simulink model "gm_uz_pmsm_model"  (R2023b)
settings: Solver=FixedStepAuto  StartTime=0.0  StopTime=0.05  RelTol=1e-3
PreLoadFcn:
  | uz_pmsm_model_init_parameter
PostLoadFcn:
  | % Import the data from Excel for a lookup table
  | FluxMapData = readtable('C:\Users\Philipp\ultrazohm\ultrazohm_sw\ip_cores\uz_pmsm_model\FluxMapData_2023-05-26_13-07-57.csv');
  | % Row indices for lookup table
  | d_current_in_d_axis = FluxMapData(8:27,1:end);
  | % Column indices for lookup table
  | q_current_in_d_axis = FluxMapData(29:48,1:end);
  | % Output values for lookup table
  | d_Flux_d_axis = FluxMapData(50:69,1:end);
undefined symbols (not defined in the file or in its folder): ad1, ad2, ad3, ad4, ad5, ad6, aq1, aq2, aq3, aq4, aq5, aq6, d_current_d_Flux, d_current_q_Flux, entkopplung_dynamic, entkopplung_linear, entkopplung_static, Fid1_Giq1, Fid2_Giq2, Flux_d, Flux_q, friction_coefficient, inertia, Ki_Bo_d, Ki_Bo_q, Kp_Bo_d, Kp_Bo_q, L_d, L_q, Ldq, parameter_nachfuerung, polepair, praediktion_entkopplung_nonlinear, psi_pm, q_current_d_Flux, q_current_q_Flux, R_1, simulate_mechanical, simulate_nonlinear_modell, simulate_open_loop, static_friction_torque, tau_sum, ts_regler
libraries: hdlmdlgenlib x21, slpidlib x6
(part 3 of 4)

== system gm_uz_pmsm_model/Current_Controller1/Entkopplungen ==
  u_q : Inport
  u_d : Inport  Port=2
  uq : Inport  Port=3
  ud : Inport  Port=4
  i_d : Inport  Port=5
  psi_d_LUT : Inport  Port=6
  psi_q_LUT : Inport  Port=7
  Ldq_LUT : Inport  Port=8
  Lqd_LUT : Inport  Port=9
  i_q : Inport  Port=10
  omega_m : Inport  Port=11
  Lineare_Entkopplung : Subsystem
  decoupling_praediktion : Subsystem
  dynamic_nonlinear_entkopplung1 : Subsystem  Commented=on
  static_nonlinear_entkopplung : Subsystem
  u_d_static : Outport
  u_q_static : Outport  Port=2
  u_d_prae : Outport  Port=3
  u_q_prae : Outport  Port=4
  u_d_lin : Outport  Port=5
  u_q_lin : Outport  Port=6
  u_d_dyn : Outport  Port=7
  u_q_dyn1 : Outport  Port=8
  wires:
  Lqd_LUT/1 -> dynamic_nonlinear_entkopplung1/6(Lqd_LUT)
  Ldq_LUT/1 -> dynamic_nonlinear_entkopplung1/5(Ldq_LUT)
  dynamic_nonlinear_entkopplung1/2(u_q) -> u_q_dyn1/1
  dynamic_nonlinear_entkopplung1/1(u_d) -> u_d_dyn/1
  decoupling_praediktion/2(u_q_entk) -> u_q_prae/1
  Lineare_Entkopplung/2(u_q) -> u_q_lin/1
  decoupling_praediktion/1(u_d_entk) -> u_d_prae/1
  static_nonlinear_entkopplung/2(u_q) -> u_q_static/1
  Lineare_Entkopplung/1(u_d) -> u_d_lin/1
  static_nonlinear_entkopplung/1(u_d) -> u_d_static/1
  u_d/1 -> decoupling_praediktion/2(u_d_1)
  uq/1 -> decoupling_praediktion/7(u_q_k)
  ud/1 -> decoupling_praediktion/6(u_d_k)
  i_q/1 -> decoupling_praediktion/3(i_q), Lineare_Entkopplung/2(i_q), dynamic_nonlinear_entkopplung1/2(i_q)
  i_d/1 -> decoupling_praediktion/1(i_d), Lineare_Entkopplung/1(i_d), dynamic_nonlinear_entkopplung1/1(i_d)
  u_q/1 -> decoupling_praediktion/4(u_q_1)
  psi_q_LUT/1 -> static_nonlinear_entkopplung/2(psi_q), decoupling_praediktion/8(psi_q), dynamic_nonlinear_entkopplung1/4(psi_q)
  omega_m/1 -> decoupling_praediktion/5(omega_m), static_nonlinear_entkopplung/3(omega_m), Lineare_Entkopplung/3(omega_m), dynamic_nonlinear_entkopplung1/7(omega_m)
  psi_d_LUT/1 -> decoupling_praediktion/9(psi_d), dynamic_nonlinear_entkopplung1/3(psi_d), static_nonlinear_entkopplung/1(psi_d)

== system gm_uz_pmsm_model/Current_Controller1/Psi_d_q1 ==
  I_d : Inport
  I_q : Inport  Port=2
  ApproxPara : Inport  Port=3
  Ldd_approx1 : Subsystem
  Lqq_approx1 : Subsystem
  psid_approx : Subsystem
  psiq_approx : Subsystem
  psi_d : Outport
  Ldd : Outport  Port=2
  psi_q : Outport  Port=3
  Lqq : Outport  Port=4
  wires:
  ApproxPara/1 -> Lqq_approx1/3(FittingParameters), psid_approx/3(FittingParameters), Ldd_approx1/3(FittingParameters), psiq_approx/3(FittingParameters)
  Lqq_approx1/1(Lqq) -> Lqq/1  "Lqq"
  Ldd_approx1/1(Ldd) -> Ldd/1  "Ldd"
  psiq_approx/2(psid_cross_s1_integrated) -> Lqq_approx1/1(psid_cross_s1_integrated)
  I_d/1 -> psiq_approx/1(Id), psid_approx/1(Id), Ldd_approx1/2(Id)
  psid_approx/2(psiq_cross_s1_integrated) -> Ldd_approx1/1(psiq_cross_s1_integrated)
  I_q/1 -> psiq_approx/2(Iq), Lqq_approx1/2(Iq), psid_approx/2(Iq)
  psiq_approx/1(psiq) -> psi_q/1  "psi_q"
  psid_approx/1(psid) -> psi_d/1  "psi_d"

== system gm_uz_pmsm_model/Current_Controller1/Reglernachführung ==
  Flag : Inport
  Ldd : Inport  Port=2
  Lqq : Inport  Port=3
  Constant : Constant  Value=1/(2*tau_sum)
  Constant1 : Constant  Value=R_1
  Constant2 : Constant  Value=L_d
  Constant3 : Constant  Value=L_q
  Product : Product
  Product1 : Product
  Product2 : Product
  Rate Transition1 : RateTransition  OutPortSampleTime=ts_regler
  Rate Transition12 : RateTransition  OutPortSampleTime=ts_regler
  Switch : Switch  Criteria=u2 > Threshold  SaturateOnIntegerOverflow=off  InputSameDT=off  OutDataTypeStr=Inherit: Same as first input
  Switch1 : Switch  Criteria=u2 > Threshold  SaturateOnIntegerOverflow=off  InputSameDT=off  OutDataTypeStr=Inherit: Same as first input
  K_p_d : Outport
  K_p_q : Outport  Port=2
  K_I : Outport  Port=3
  wires:
  Constant1/1 -> Rate Transition1/1  "u_q"
  Lqq/1 -> Switch1/1  "Lqq"
  Ldd/1 -> Switch/1  "Ldd"
  Switch1/1 -> Product1/2
  Constant3/1 -> Switch1/3
  Switch/1 -> Product/1
  Constant2/1 -> Switch/3
  Flag/1 -> Switch1/2, Switch/2
  Rate Transition1/1 -> Product2/2  "id_regler"
  Rate Transition12/1 -> Product/2, Product1/1, Product2/1  "id_regler"
  Product2/1 -> K_I/1
  Product1/1 -> K_p_q/1
  Product/1 -> K_p_d/1
  Constant/1 -> Rate Transition12/1

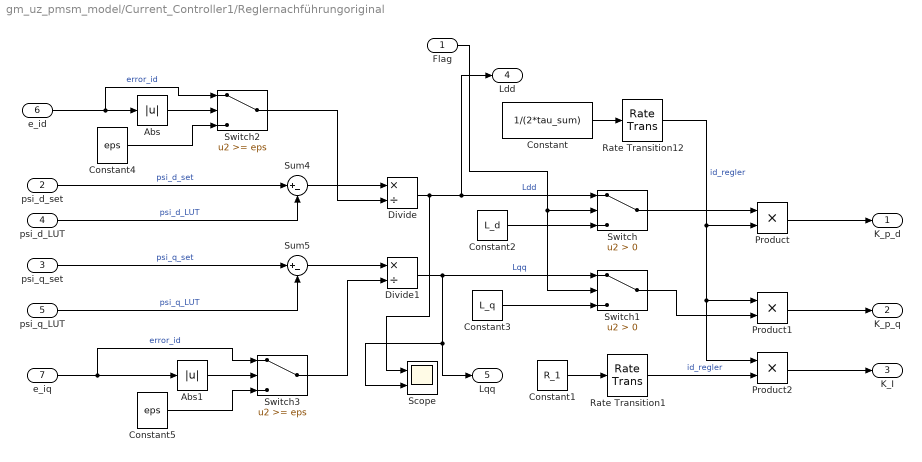
== system gm_uz_pmsm_model/Current_Controller1/Reglernachführungoriginal ==
  Flag : Inport
  psi_d_set : Inport  Port=2
  psi_q_set : Inport  Port=3
  psi_d_LUT : Inport  Port=4
  psi_q_LUT : Inport  Port=5
  e_id : Inport  Port=6
  e_iq : Inport  Port=7
  Abs : Abs  SaturateOnIntegerOverflow=off
  Abs1 : Abs  SaturateOnIntegerOverflow=off
  Constant : Constant  Value=1/(2*tau_sum)
  Constant1 : Constant  Value=R_1
  Constant2 : Constant  Value=L_d
  Constant3 : Constant  Value=L_q
  Constant4 : Constant  Value=eps  SampleTime=ts_regler
  Constant5 : Constant  Value=eps  SampleTime=ts_regler
  Divide : Product  Inputs=*/
  Divide1 : Product  Inputs=*/
  Product : Product
  Product1 : Product
  Product2 : Product
  Rate Transition1 : RateTransition  OutPortSampleTime=ts_regler
  Rate Transition12 : RateTransition  OutPortSampleTime=ts_regler
  Scope : Scope  NumInputPorts=2
  Sum4 : Sum  Inputs=|+-
  Sum5 : Sum  Inputs=|+-
  Switch : Switch  Criteria=u2 > Threshold  SaturateOnIntegerOverflow=off  InputSameDT=off
  Switch1 : Switch  Criteria=u2 > Threshold  SaturateOnIntegerOverflow=off  InputSameDT=off
  Switch2 : Switch  Threshold=eps  SaturateOnIntegerOverflow=off  InputSameDT=off
  Switch3 : Switch  Threshold=eps  SaturateOnIntegerOverflow=off  InputSameDT=off
  K_p_d : Outport
  K_p_q : Outport  Port=2
  K_I : Outport  Port=3
  Ldd : Outport  Port=4
  Lqq : Outport  Port=5
  wires:
  Constant5/1 -> Switch3/3
  Abs1/1 -> Switch3/2
  Switch3/1 -> Divide1/2
  e_iq/1 -> Abs1/1, Switch3/1  "error_id"
  Switch2/1 -> Divide/2
  Abs/1 -> Switch2/2
  Constant4/1 -> Switch2/3
  e_id/1 -> Abs/1, Switch2/1  "error_id"
  Divide1/1 -> Switch1/1, Lqq/1, Scope/2  "Lqq"
  Divide/1 -> Switch/1, Ldd/1, Scope/1  "Ldd"
  psi_q_set/1 -> Sum5/1  "psi_q_set"
  psi_d_set/1 -> Sum4/1  "psi_d_set"
  psi_d_LUT/1 -> Sum4/2  "psi_d_LUT"
  Sum5/1 -> Divide1/1
  psi_q_LUT/1 -> Sum5/2  "psi_q_LUT"
  Sum4/1 -> Divide/1
  Switch1/1 -> Product1/2
  Constant3/1 -> Switch1/3
  Switch/1 -> Product/1
  Constant2/1 -> Switch/3
  Flag/1 -> Switch1/2, Switch/2
  Rate Transition1/1 -> Product2/2  "id_regler"
  Rate Transition12/1 -> Product/2, Product1/1, Product2/1  "id_regler"
  Constant1/1 -> Rate Transition1/1
  Product2/1 -> K_I/1
  Product1/1 -> K_p_q/1
  Product/1 -> K_p_d/1
  Constant/1 -> Rate Transition12/1

== system gm_uz_pmsm_model/Current_Controller_With_FluxMaps_OLD1/Entkopplung_flags ==
  u_d_static : Inport
  u_q_static : Inport  Port=2
  u_d_praed : Inport  Port=3
  u_q_praed : Inport  Port=4
  u_d_lin : Inport  Port=5
  u_q_lin : Inport  Port=6
  u_d_dyn : Inport  Port=7
  u_q_dyn : Inport  Port=8
  0 : Constant  Value=0
  Switch{1..8} (8 alike) : Switch  Criteria=u2 > Threshold  SaturateOnIntegerOverflow=off  InputSameDT=off
  entkopplung_dynamic : Constant  Value=entkopplung_dynamic
  entkopplung_linear : Constant  Value=entkopplung_linear
  entkopplung_preadiktion : Constant  Value=praediktion_entkopplung_nonlinear
  entkopplung_static : Constant  Value=entkopplung_static
  u_d_entk : Outport
  u_q_entk : Outport  Port=2
  wires:
  Switch7/1 -> Switch5/3
  u_q_dyn/1 -> Switch8/1
  Switch8/1 -> Switch6/3
  u_d_dyn/1 -> Switch7/1
  u_q_lin/1 -> Switch6/1
  u_q_static/1 -> Switch4/1
  Switch6/1 -> Switch4/3
  0/1 -> Switch7/3, Switch8/3
  entkopplung_dynamic/1 -> Switch7/2, Switch8/2
  entkopplung_linear/1 -> Switch5/2, Switch6/2
  Switch5/1 -> Switch1/3
  u_d_lin/1 -> Switch5/1
  u_d_static/1 -> Switch1/1
  entkopplung_static/1 -> Switch1/2, Switch4/2
  u_q_praed/1 -> Switch2/1
  Switch2/1 -> u_q_entk/1
  u_d_praed/1 -> Switch3/1
  Switch1/1 -> Switch3/3
  entkopplung_preadiktion/1 -> Switch3/2, Switch2/2
  Switch4/1 -> Switch2/3
  Switch3/1 -> u_d_entk/1

== system gm_uz_pmsm_model/Current_Controller_With_FluxMaps_OLD1/Entkopplungen ==
  u_q : Inport
  u_d : Inport  Port=2
  uq : Inport  Port=3
  ud : Inport  Port=4
  i_d : Inport  Port=5
  psi_d_LUT : Inport  Port=6
  psi_q_LUT : Inport  Port=7
  Ldq_LUT : Inport  Port=8
  Lqd_LUT : Inport  Port=9
  i_q : Inport  Port=10
  omega_m : Inport  Port=11
  Lineare_Entkopplung : Subsystem
  decoupling_praediktion : Subsystem
  dynamic_nonlinear_entkopplung1 : Subsystem
  static_nonlinear_entkopplung : Subsystem
  u_d_static : Outport
  u_q_static : Outport  Port=2
  u_d_prae : Outport  Port=3
  u_q_prae : Outport  Port=4
  u_d_lin : Outport  Port=5
  u_q_lin : Outport  Port=6
  u_d_dyn : Outport  Port=7
  u_q_dyn1 : Outport  Port=8
  wires:
  Lqd_LUT/1 -> dynamic_nonlinear_entkopplung1/6(Lqd_LUT)
  Ldq_LUT/1 -> dynamic_nonlinear_entkopplung1/5(Ldq_LUT)
  dynamic_nonlinear_entkopplung1/2(u_q) -> u_q_dyn1/1
  dynamic_nonlinear_entkopplung1/1(u_d) -> u_d_dyn/1
  decoupling_praediktion/2(u_q_entk) -> u_q_prae/1
  Lineare_Entkopplung/2(u_q) -> u_q_lin/1
  decoupling_praediktion/1(u_d_entk) -> u_d_prae/1
  static_nonlinear_entkopplung/2(u_q) -> u_q_static/1
  Lineare_Entkopplung/1(u_d) -> u_d_lin/1
  static_nonlinear_entkopplung/1(u_d) -> u_d_static/1
  u_d/1 -> decoupling_praediktion/2(u_d_1)
  uq/1 -> decoupling_praediktion/7(u_q_k)
  ud/1 -> decoupling_praediktion/6(u_d_k)
  i_q/1 -> decoupling_praediktion/3(i_q), Lineare_Entkopplung/2(i_q), dynamic_nonlinear_entkopplung1/2(i_q)
  i_d/1 -> decoupling_praediktion/1(i_d), Lineare_Entkopplung/1(i_d), dynamic_nonlinear_entkopplung1/1(i_d)
  u_q/1 -> decoupling_praediktion/4(u_q_1)
  psi_q_LUT/1 -> static_nonlinear_entkopplung/2(psi_q), decoupling_praediktion/8(psi_q), dynamic_nonlinear_entkopplung1/4(psi_q)
  omega_m/1 -> decoupling_praediktion/5(omega_m), static_nonlinear_entkopplung/3(omega_m), Lineare_Entkopplung/3(omega_m), dynamic_nonlinear_entkopplung1/7(omega_m)
  psi_d_LUT/1 -> decoupling_praediktion/9(psi_d), dynamic_nonlinear_entkopplung1/3(psi_d), static_nonlinear_entkopplung/1(psi_d)

== system gm_uz_pmsm_model/Current_Controller_With_FluxMaps_OLD1/Psi_d_q ==
  I_d_set : Inport
  I_d : Inport  Port=2
  I_q_set : Inport  Port=3
  I_q : Inport  Port=4
  Flux_d Lookup Table : Lookup_n-D  BreakpointsForDimension1=d_current_d_Flux  BreakpointsForDimension2=q_current_d_Flux  BreakpointsForDimension3=[5, 7]  Table=Flux_d  InternalRulePriority=Speed  RndMeth=Simplest
      settings: InputPortMap=u0,u1
  Flux_d Lookup Table1 : Lookup_n-D  BreakpointsForDimension1=d_current_d_Flux  BreakpointsForDimension2=q_current_d_Flux  BreakpointsForDimension3=[5, 7]  Table=Flux_d  InternalRulePriority=Speed  RndMeth=Simplest
      settings: InputPortMap=u0,u1
  Flux_q Lookup Table1 : Lookup_n-D  BreakpointsForDimension1=d_current_q_Flux  BreakpointsForDimension2=q_current_q_Flux  BreakpointsForDimension3=[5, 7]  Table=Flux_q  InternalRulePriority=Speed  RndMeth=Simplest
      settings: InputPortMap=u0,u1
  Flux_q Lookup Table2 : Lookup_n-D  BreakpointsForDimension1=d_current_q_Flux  BreakpointsForDimension2=q_current_q_Flux  BreakpointsForDimension3=[5, 7]  Table=Flux_q  InternalRulePriority=Speed  RndMeth=Simplest
      settings: InputPortMap=u0,u1
  Ldq Lookup Table : Lookup_n-D  BreakpointsForDimension1=d_current_q_Flux  BreakpointsForDimension2=q_current_q_Flux  BreakpointsForDimension3=[5, 7]  Table=Ldq  ExtrapMethod=Clip  UseLastTableValue=on  InternalRulePriority=Speed  OutDataTypeStr=Inherit: Inherit from 'Table data'  RndMeth=Simplest
      settings: InputPortMap=u0,u1
  Lqd Lookup Table1 : Lookup_n-D  BreakpointsForDimension1=d_current_q_Flux  BreakpointsForDimension2=q_current_q_Flux  BreakpointsForDimension3=[5, 7]  Table=Ldq  ExtrapMethod=Clip  UseLastTableValue=on  InternalRulePriority=Speed  OutDataTypeStr=Inherit: Inherit from 'Table data'  RndMeth=Simplest
      settings: InputPortMap=u0,u1
  Scope : Scope  NumInputPorts=4
  psi_d_set : Outport
  psi_q_set : Outport  Port=2
  psi_d_LUT : Outport  Port=3
  psi_q_LUT : Outport  Port=4
  Ldq_LUT : Outport  Port=5
  Lqd_LUT : Outport  Port=6
  wires:
  I_q/1 -> Flux_d Lookup Table/2, Flux_d Lookup Table1/2, Flux_q Lookup Table1/2, Ldq Lookup Table/2, Lqd Lookup Table1/2, Scope/4
  I_d/1 -> Flux_d Lookup Table/1, Flux_q Lookup Table1/1, Ldq Lookup Table/1, Lqd Lookup Table1/1, Flux_q Lookup Table2/1, Scope/3
  Lqd Lookup Table1/1 -> Lqd_LUT/1  "Ldq_Karte"
  Ldq Lookup Table/1 -> Ldq_LUT/1  "Ldq_Karte"
  Flux_q Lookup Table1/1 -> psi_q_LUT/1  "psi_q_controller"
  Flux_d Lookup Table/1 -> psi_d_LUT/1  "psi_d_controller"
  Flux_q Lookup Table2/1 -> psi_q_set/1  "psi_q_set"
  Flux_d Lookup Table1/1 -> psi_d_set/1  "psi_d_set"
  I_q_set/1 -> Flux_q Lookup Table2/2, Scope/2
  I_d_set/1 -> Flux_d Lookup Table1/1, Scope/1

== system gm_uz_pmsm_model/Current_Controller_With_FluxMaps_OLD1/Psi_d_q1 ==
  I_d_set : Inport
  I_d : Inport  Port=2
  I_q_set : Inport  Port=3
  I_q : Inport  Port=4
  Flux_d Lookup Table : Lookup_n-D  BreakpointsForDimension1=d_current_d_Flux  BreakpointsForDimension2=q_current_d_Flux  BreakpointsForDimension3=[5, 7]  Table=Flux_d  InternalRulePriority=Speed  RndMeth=Simplest
      settings: InputPortMap=u0,u1
  Flux_d Lookup Table1 : Lookup_n-D  BreakpointsForDimension1=d_current_d_Flux  BreakpointsForDimension2=q_current_d_Flux  BreakpointsForDimension3=[5, 7]  Table=Flux_d  InternalRulePriority=Speed  RndMeth=Simplest
      settings: InputPortMap=u0,u1
  Flux_q Lookup Table1 : Lookup_n-D  BreakpointsForDimension1=d_current_q_Flux  BreakpointsForDimension2=q_current_q_Flux  BreakpointsForDimension3=[5, 7]  Table=Flux_q  InternalRulePriority=Speed  RndMeth=Simplest
      settings: InputPortMap=u0,u1
  Flux_q Lookup Table2 : Lookup_n-D  BreakpointsForDimension1=d_current_q_Flux  BreakpointsForDimension2=q_current_q_Flux  BreakpointsForDimension3=[5, 7]  Table=Flux_q  InternalRulePriority=Speed  RndMeth=Simplest
      settings: InputPortMap=u0,u1
  Ldq Lookup Table : Lookup_n-D  BreakpointsForDimension1=d_current_q_Flux  BreakpointsForDimension2=q_current_q_Flux  BreakpointsForDimension3=[5, 7]  Table=Ldq  ExtrapMethod=Clip  UseLastTableValue=on  InternalRulePriority=Speed  OutDataTypeStr=Inherit: Inherit from 'Table data'  RndMeth=Simplest
      settings: InputPortMap=u0,u1
  Lqd Lookup Table1 : Lookup_n-D  BreakpointsForDimension1=d_current_q_Flux  BreakpointsForDimension2=q_current_q_Flux  BreakpointsForDimension3=[5, 7]  Table=Ldq  ExtrapMethod=Clip  UseLastTableValue=on  InternalRulePriority=Speed  OutDataTypeStr=Inherit: Inherit from 'Table data'  RndMeth=Simplest
      settings: InputPortMap=u0,u1
  psi_d_set : Outport
  psi_q_set : Outport  Port=2
  psi_d_LUT : Outport  Port=3
  psi_q_LUT : Outport  Port=4
  Ldq_LUT : Outport  Port=5
  Lqd_LUT : Outport  Port=6
  wires:
  I_q/1 -> Flux_d Lookup Table/2, Flux_d Lookup Table1/2, Flux_q Lookup Table1/2, Ldq Lookup Table/2, Lqd Lookup Table1/2
  I_d/1 -> Flux_d Lookup Table/1, Flux_q Lookup Table1/1, Ldq Lookup Table/1, Lqd Lookup Table1/1, Flux_q Lookup Table2/1
  Lqd Lookup Table1/1 -> Lqd_LUT/1  "Ldq_Karte"
  Ldq Lookup Table/1 -> Ldq_LUT/1  "Ldq_Karte"
  Flux_q Lookup Table1/1 -> psi_q_LUT/1  "psi_q_controller"
  Flux_d Lookup Table/1 -> psi_d_LUT/1  "psi_d_controller"
  Flux_q Lookup Table2/1 -> psi_q_set/1  "psi_q_set"
  Flux_d Lookup Table1/1 -> psi_d_set/1  "psi_d_set"
  I_q_set/1 -> Flux_q Lookup Table2/2
  I_d_set/1 -> Flux_d Lookup Table1/1

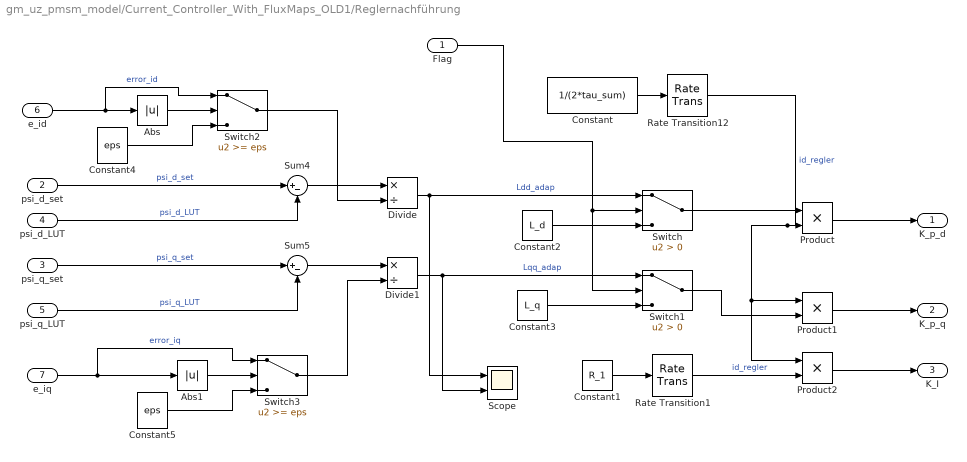
== system gm_uz_pmsm_model/Current_Controller_With_FluxMaps_OLD1/Reglernachführung ==
  Flag : Inport
  psi_d_set : Inport  Port=2
  psi_q_set : Inport  Port=3
  psi_d_LUT : Inport  Port=4
  psi_q_LUT : Inport  Port=5
  e_id : Inport  Port=6
  e_iq : Inport  Port=7
  Abs : Abs  SaturateOnIntegerOverflow=off
  Abs1 : Abs  SaturateOnIntegerOverflow=off
  Constant : Constant  Value=1/(2*tau_sum)
  Constant1 : Constant  Value=R_1
  Constant2 : Constant  Value=L_d
  Constant3 : Constant  Value=L_q
  Constant4 : Constant  Value=eps  SampleTime=ts_regler
  Constant5 : Constant  Value=eps  SampleTime=ts_regler
  Divide : Product  Inputs=*/
  Divide1 : Product  Inputs=*/
  Product : Product
  Product1 : Product
  Product2 : Product
  Rate Transition1 : RateTransition  OutPortSampleTime=ts_regler
  Rate Transition12 : RateTransition  OutPortSampleTime=ts_regler
  Scope : Scope  NumInputPorts=2
  Sum4 : Sum  Inputs=|+-
  Sum5 : Sum  Inputs=|+-
  Switch : Switch  Criteria=u2 > Threshold  SaturateOnIntegerOverflow=off  InputSameDT=off
  Switch1 : Switch  Criteria=u2 > Threshold  SaturateOnIntegerOverflow=off  InputSameDT=off
  Switch2 : Switch  Threshold=eps  SaturateOnIntegerOverflow=off  InputSameDT=off
  Switch3 : Switch  Threshold=eps  SaturateOnIntegerOverflow=off  InputSameDT=off
  K_p_d : Outport
  K_p_q : Outport  Port=2
  K_I : Outport  Port=3
  wires:
  Constant5/1 -> Switch3/3
  Abs1/1 -> Switch3/2
  Switch3/1 -> Divide1/2
  e_iq/1 -> Abs1/1, Switch3/1  "error_iq"
  Switch2/1 -> Divide/2
  Abs/1 -> Switch2/2
  Constant4/1 -> Switch2/3
  e_id/1 -> Abs/1, Switch2/1  "error_id"
  Divide1/1 -> Switch1/1, Scope/2  "Lqq_adap"
  Divide/1 -> Switch/1, Scope/1  "Ldd_adap"
  psi_q_set/1 -> Sum5/1  "psi_q_set"
  psi_d_set/1 -> Sum4/1  "psi_d_set"
  psi_d_LUT/1 -> Sum4/2  "psi_d_LUT"
  Sum5/1 -> Divide1/1
  psi_q_LUT/1 -> Sum5/2  "psi_q_LUT"
  Sum4/1 -> Divide/1
  Switch1/1 -> Product1/2
  Constant3/1 -> Switch1/3
  Switch/1 -> Product/1
  Constant2/1 -> Switch/3
  Flag/1 -> Switch1/2, Switch/2
  Rate Transition1/1 -> Product2/2  "id_regler"
  Rate Transition12/1 -> Product/2, Product1/1, Product2/1  "id_regler"
  Constant1/1 -> Rate Transition1/1
  Product2/1 -> K_I/1
  Product1/1 -> K_p_q/1
  Product/1 -> K_p_d/1
  Constant/1 -> Rate Transition12/1

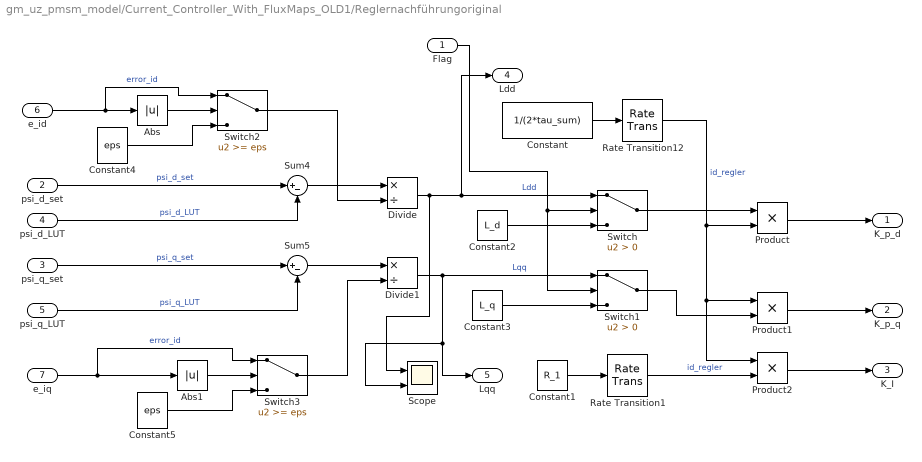
== system gm_uz_pmsm_model/Current_Controller_With_FluxMaps_OLD1/Reglernachführungoriginal ==
  Flag : Inport
  psi_d_set : Inport  Port=2
  psi_q_set : Inport  Port=3
  psi_d_LUT : Inport  Port=4
  psi_q_LUT : Inport  Port=5
  e_id : Inport  Port=6
  e_iq : Inport  Port=7
  Abs : Abs  SaturateOnIntegerOverflow=off
  Abs1 : Abs  SaturateOnIntegerOverflow=off
  Constant : Constant  Value=1/(2*tau_sum)
  Constant1 : Constant  Value=R_1
  Constant2 : Constant  Value=L_d
  Constant3 : Constant  Value=L_q
  Constant4 : Constant  Value=eps  SampleTime=ts_regler
  Constant5 : Constant  Value=eps  SampleTime=ts_regler
  Divide : Product  Inputs=*/
  Divide1 : Product  Inputs=*/
  Product : Product
  Product1 : Product
  Product2 : Product
  Rate Transition1 : RateTransition  OutPortSampleTime=ts_regler
  Rate Transition12 : RateTransition  OutPortSampleTime=ts_regler
  Scope : Scope  NumInputPorts=2
  Sum4 : Sum  Inputs=|+-
  Sum5 : Sum  Inputs=|+-
  Switch : Switch  Criteria=u2 > Threshold  SaturateOnIntegerOverflow=off  InputSameDT=off
  Switch1 : Switch  Criteria=u2 > Threshold  SaturateOnIntegerOverflow=off  InputSameDT=off
  Switch2 : Switch  Threshold=eps  SaturateOnIntegerOverflow=off  InputSameDT=off
  Switch3 : Switch  Threshold=eps  SaturateOnIntegerOverflow=off  InputSameDT=off
  K_p_d : Outport
  K_p_q : Outport  Port=2
  K_I : Outport  Port=3
  Ldd : Outport  Port=4
  Lqq : Outport  Port=5
  wires:
  Constant5/1 -> Switch3/3
  Abs1/1 -> Switch3/2
  Switch3/1 -> Divide1/2
  e_iq/1 -> Abs1/1, Switch3/1  "error_id"
  Switch2/1 -> Divide/2
  Abs/1 -> Switch2/2
  Constant4/1 -> Switch2/3
  e_id/1 -> Abs/1, Switch2/1  "error_id"
  Divide1/1 -> Switch1/1, Lqq/1, Scope/2  "Lqq"
  Divide/1 -> Switch/1, Ldd/1, Scope/1  "Ldd"
  psi_q_set/1 -> Sum5/1  "psi_q_set"
  psi_d_set/1 -> Sum4/1  "psi_d_set"
  psi_d_LUT/1 -> Sum4/2  "psi_d_LUT"
  Sum5/1 -> Divide1/1
  psi_q_LUT/1 -> Sum5/2  "psi_q_LUT"
  Sum4/1 -> Divide/1
  Switch1/1 -> Product1/2
  Constant3/1 -> Switch1/3
  Switch/1 -> Product/1
  Constant2/1 -> Switch/3
  Flag/1 -> Switch1/2, Switch/2
  Rate Transition1/1 -> Product2/2  "id_regler"
  Rate Transition12/1 -> Product/2, Product1/1, Product2/1  "id_regler"
  Constant1/1 -> Rate Transition1/1
  Product2/1 -> K_I/1
  Product1/1 -> K_p_q/1
  Product/1 -> K_p_d/1
  Constant/1 -> Rate Transition12/1

== system gm_uz_pmsm_model/uz_pmsm_model/Abs ==
  In1 : Inport
  Abs : Abs  SampleTime=1e-08  OutDataTypeStr=single  SaturateOnIntegerOverflow=off
  Out1 : Outport
  wires:
  In1/1 -> Abs/1
  Abs/1 -> Out1/1

== system gm_uz_pmsm_model/uz_pmsm_model/Divide ==
  In1 : Inport
  In2 : Inport  Port=2
  Divide : Product  Inputs=**  OutDataTypeStr=single  SampleTime=1e-08
  Divide_pd1 : Delay  DelayLength=6
  Out1 : Outport
  wires:
  In1/1 -> Divide/1
  In2/1 -> Divide/2
  Divide/1 -> Divide_pd1/1
  Divide_pd1/1 -> Out1/1

== system gm_uz_pmsm_model/uz_pmsm_model/Divide1 ==
  In1 : Inport
  In2 : Inport  Port=2
  Divide1 : Product  Inputs=*/  OutDataTypeStr=single  SampleTime=1e-08
  Divide1_pd1 : Delay  DelayLength=17
  Out1 : Outport
  wires:
  In1/1 -> Divide1/1
  In2/1 -> Divide1/2
  Divide1/1 -> Divide1_pd1/1
  Divide1_pd1/1 -> Out1/1

== system gm_uz_pmsm_model/uz_pmsm_model/Divide_recip ==
  In1 : Inport
  Divide_recip : Math  Operator=reciprocal  SampleTime=1e-08
  Divide_recip_pd1 : Delay  DelayLength=16
  Out1 : Outport
  wires:
  In1/1 -> Divide_recip/1
  Divide_recip/1 -> Divide_recip_pd1/1
  Divide_recip_pd1/1 -> Out1/1

== system gm_uz_pmsm_model/uz_pmsm_model/Factor ==
  In1 : Inport
  In2 : Inport  Port=2
  Factor : Product  Inputs=**  OutDataTypeStr=single  SampleTime=1e-08
  Factor_pd1 : Delay  DelayLength=6
  Out1 : Outport
  wires:
  In1/1 -> Factor/1
  In2/1 -> Factor/2
  Factor/1 -> Factor_pd1/1
  Factor_pd1/1 -> Out1/1

== system gm_uz_pmsm_model/uz_pmsm_model/Gain ==
  In1 : Inport
  In2 : Inport  Port=2
  Gain : Product  Inputs=**  OutDataTypeStr=single  SampleTime=1e-08
  Gain_pd1 : Delay  DelayLength=6
  Out1 : Outport
  wires:
  In1/1 -> Gain/1
  In2/1 -> Gain/2
  Gain/1 -> Gain_pd1/1
  Gain_pd1/1 -> Out1/1

== system gm_uz_pmsm_model/uz_pmsm_model/Gain7 ==
  In1 : Inport
  In2 : Inport  Port=2
  Gain7 : Product  Inputs=**  OutDataTypeStr=single  SampleTime=1e-08
  Gain7_pd1 : Delay  DelayLength=6
  Out1 : Outport
  wires:
  In1/1 -> Gain7/1
  In2/1 -> Gain7/2
  Gain7/1 -> Gain7_pd1/1
  Gain7_pd1/1 -> Out1/1

== system gm_uz_pmsm_model/uz_pmsm_model/Gain71 ==
  In1 : Inport
  In2 : Inport  Port=2
  Gain71 : Product  Inputs=**  OutDataTypeStr=single  SampleTime=1e-08
  Gain71_pd1 : Delay  DelayLength=6
  Out1 : Outport
  wires:
  In1/1 -> Gain71/1
  In2/1 -> Gain71/2
  Gain71/1 -> Gain71_pd1/1
  Gain71_pd1/1 -> Out1/1

== system gm_uz_pmsm_model/uz_pmsm_model/Gain_unaryminus ==
  In1 : Inport
  Gain_unaryminus : UnaryMinus  SampleTime=1e-08
  Out1 : Outport
  wires:
  In1/1 -> Gain_unaryminus/1
  Gain_unaryminus/1 -> Out1/1

== system gm_uz_pmsm_model/uz_pmsm_model/Gain_unaryminus1 ==
  In1 : Inport
  Gain_unaryminus1 : UnaryMinus  SampleTime=1e-08
  Out1 : Outport
  wires:
  In1/1 -> Gain_unaryminus1/1
  Gain_unaryminus1/1 -> Out1/1

== system gm_uz_pmsm_model/uz_pmsm_model/Log ==
  In1 : Inport
  Log : Math  Operator=log  SampleTime=1e-08
  Log_pd1 : Delay  DelayLength=20
  Out1 : Outport
  wires:
  In1/1 -> Log/1
  Log/1 -> Log_pd1/1
  Log_pd1/1 -> Out1/1

== system gm_uz_pmsm_model/uz_pmsm_model/Log1 ==
  In1 : Inport
  Log1 : Math  Operator=log  SampleTime=1e-08
  Log1_pd1 : Delay  DelayLength=20
  Out1 : Outport
  wires:
  In1/1 -> Log1/1
  Log1/1 -> Log1_pd1/1
  Log1_pd1/1 -> Out1/1

== system gm_uz_pmsm_model/uz_pmsm_model/Log11 ==
  In1 : Inport
  Log11 : Math  Operator=log  SampleTime=1e-08
  Log11_pd1 : Delay  DelayLength=20
  Out1 : Outport
  wires:
  In1/1 -> Log11/1
  Log11/1 -> Log11_pd1/1
  Log11_pd1/1 -> Out1/1

== system gm_uz_pmsm_model/uz_pmsm_model/Log2 ==
  In1 : Inport
  Log2 : Math  Operator=log  SampleTime=1e-08
  Log2_pd1 : Delay  DelayLength=20
  Out1 : Outport
  wires:
  In1/1 -> Log2/1
  Log2/1 -> Log2_pd1/1
  Log2_pd1/1 -> Out1/1

== system gm_uz_pmsm_model/uz_pmsm_model/Product ==
  In1 : Inport
  In2 : Inport  Port=2
  Product : Product  Inputs=**  OutDataTypeStr=single  SampleTime=1e-08
  Product_pd1 : Delay  DelayLength=6
  Out1 : Outport
  wires:
  In1/1 -> Product/1
  In2/1 -> Product/2
  Product/1 -> Product_pd1/1
  Product_pd1/1 -> Out1/1

== system gm_uz_pmsm_model/uz_pmsm_model/Product1 ==
  In1 : Inport
  In2 : Inport  Port=2
  Product1 : Product  Inputs=**  OutDataTypeStr=single  SampleTime=1e-08
  Product1_pd1 : Delay  DelayLength=6
  Out1 : Outport
  wires:
  In1/1 -> Product1/1
  In2/1 -> Product1/2
  Product1/1 -> Product1_pd1/1
  Product1_pd1/1 -> Out1/1

== system gm_uz_pmsm_model/uz_pmsm_model/Product10 ==
  In1 : Inport
  In2 : Inport  Port=2
  Product10 : Product  Inputs=**  OutDataTypeStr=single  SampleTime=1e-08
  Product10_pd1 : Delay  DelayLength=6
  Out1 : Outport
  wires:
  In1/1 -> Product10/1
  In2/1 -> Product10/2
  Product10/1 -> Product10_pd1/1
  Product10_pd1/1 -> Out1/1

== system gm_uz_pmsm_model/uz_pmsm_model/Product101 ==
  In1 : Inport
  In2 : Inport  Port=2
  Product101 : Product  Inputs=**  OutDataTypeStr=single  SampleTime=1e-08
  Product101_pd1 : Delay  DelayLength=6
  Out1 : Outport
  wires:
  In1/1 -> Product101/1
  In2/1 -> Product101/2
  Product101/1 -> Product101_pd1/1
  Product101_pd1/1 -> Out1/1

== system gm_uz_pmsm_model/uz_pmsm_model/Product102 ==
  In1 : Inport
  In2 : Inport  Port=2
  Product102 : Product  Inputs=**  OutDataTypeStr=single  SampleTime=1e-08
  Product102_pd1 : Delay  DelayLength=6
  Out1 : Outport
  wires:
  In1/1 -> Product102/1
  In2/1 -> Product102/2
  Product102/1 -> Product102_pd1/1
  Product102_pd1/1 -> Out1/1

== system gm_uz_pmsm_model/uz_pmsm_model/Product103 ==
  In1 : Inport
  In2 : Inport  Port=2
  Product103 : Product  Inputs=**  OutDataTypeStr=single  SampleTime=1e-08
  Product103_pd1 : Delay  DelayLength=6
  Out1 : Outport
  wires:
  In1/1 -> Product103/1
  In2/1 -> Product103/2
  Product103/1 -> Product103_pd1/1
  Product103_pd1/1 -> Out1/1

== system gm_uz_pmsm_model/uz_pmsm_model/Product104 ==
  In1 : Inport
  In2 : Inport  Port=2
  Product104 : Product  Inputs=**  OutDataTypeStr=single  SampleTime=1e-08
  Product104_pd1 : Delay  DelayLength=6
  Out1 : Outport
  wires:
  In1/1 -> Product104/1
  In2/1 -> Product104/2
  Product104/1 -> Product104_pd1/1
  Product104_pd1/1 -> Out1/1

== system gm_uz_pmsm_model/uz_pmsm_model/Product11 ==
  In1 : Inport
  In2 : Inport  Port=2
  Product11 : Product  Inputs=**  OutDataTypeStr=single  SampleTime=1e-08
  Product11_pd1 : Delay  DelayLength=6
  Out1 : Outport
  wires:
  In1/1 -> Product11/1
  In2/1 -> Product11/2
  Product11/1 -> Product11_pd1/1
  Product11_pd1/1 -> Out1/1

== system gm_uz_pmsm_model/uz_pmsm_model/Product110 ==
  In1 : Inport
  In2 : Inport  Port=2
  Product110 : Product  Inputs=**  OutDataTypeStr=single  SampleTime=1e-08
  Product110_pd1 : Delay  DelayLength=6
  Out1 : Outport
  wires:
  In1/1 -> Product110/1
  In2/1 -> Product110/2
  Product110/1 -> Product110_pd1/1
  Product110_pd1/1 -> Out1/1

== system gm_uz_pmsm_model/uz_pmsm_model/Product111 ==
  In1 : Inport
  In2 : Inport  Port=2
  Product111 : Product  Inputs=**  OutDataTypeStr=single  SampleTime=1e-08
  Product111_pd1 : Delay  DelayLength=6
  Out1 : Outport
  wires:
  In1/1 -> Product111/1
  In2/1 -> Product111/2
  Product111/1 -> Product111_pd1/1
  Product111_pd1/1 -> Out1/1

== system gm_uz_pmsm_model/uz_pmsm_model/Product12 ==
  In1 : Inport
  In2 : Inport  Port=2
  Product12 : Product  Inputs=**  OutDataTypeStr=single  SampleTime=1e-08
  Product12_pd1 : Delay  DelayLength=6
  Out1 : Outport
  wires:
  In1/1 -> Product12/1
  In2/1 -> Product12/2
  Product12/1 -> Product12_pd1/1
  Product12_pd1/1 -> Out1/1

== system gm_uz_pmsm_model/uz_pmsm_model/Product121 ==
  In1 : Inport
  In2 : Inport  Port=2
  Product121 : Product  Inputs=**  OutDataTypeStr=single  SampleTime=1e-08
  Product121_pd1 : Delay  DelayLength=6
  Out1 : Outport
  wires:
  In1/1 -> Product121/1
  In2/1 -> Product121/2
  Product121/1 -> Product121_pd1/1
  Product121_pd1/1 -> Out1/1

== system gm_uz_pmsm_model/uz_pmsm_model/Product122 ==
  In1 : Inport
  In2 : Inport  Port=2
  Product122 : Product  Inputs=**  OutDataTypeStr=single  SampleTime=1e-08
  Product122_pd1 : Delay  DelayLength=6
  Out1 : Outport
  wires:
  In1/1 -> Product122/1
  In2/1 -> Product122/2
  Product122/1 -> Product122_pd1/1
  Product122_pd1/1 -> Out1/1

== system gm_uz_pmsm_model/uz_pmsm_model/Product13 ==
  In1 : Inport
  In2 : Inport  Port=2
  Product13 : Product  Inputs=**  OutDataTypeStr=single  SampleTime=1e-08
  Product13_pd1 : Delay  DelayLength=6
  Out1 : Outport
  wires:
  In1/1 -> Product13/1
  In2/1 -> Product13/2
  Product13/1 -> Product13_pd1/1
  Product13_pd1/1 -> Out1/1

== system gm_uz_pmsm_model/uz_pmsm_model/Product131 ==
  In1 : Inport
  In2 : Inport  Port=2
  Product131 : Product  Inputs=**  OutDataTypeStr=single  SampleTime=1e-08
  Product131_pd1 : Delay  DelayLength=6
  Out1 : Outport
  wires:
  In1/1 -> Product131/1
  In2/1 -> Product131/2
  Product131/1 -> Product131_pd1/1
  Product131_pd1/1 -> Out1/1

== system gm_uz_pmsm_model/uz_pmsm_model/Product14 ==
  In1 : Inport
  In2 : Inport  Port=2
  Product14 : Product  Inputs=**  OutDataTypeStr=single  SampleTime=1e-08
  Product14_pd1 : Delay  DelayLength=6
  Out1 : Outport
  wires:
  In1/1 -> Product14/1
  In2/1 -> Product14/2
  Product14/1 -> Product14_pd1/1
  Product14_pd1/1 -> Out1/1

== system gm_uz_pmsm_model/uz_pmsm_model/Product141 ==
  In1 : Inport
  In2 : Inport  Port=2
  Product141 : Product  Inputs=**  OutDataTypeStr=single  SampleTime=1e-08
  Product141_pd1 : Delay  DelayLength=6
  Out1 : Outport
  wires:
  In1/1 -> Product141/1
  In2/1 -> Product141/2
  Product141/1 -> Product141_pd1/1
  Product141_pd1/1 -> Out1/1

== system gm_uz_pmsm_model/uz_pmsm_model/Product142 ==
  In1 : Inport
  In2 : Inport  Port=2
  Product142 : Product  Inputs=**  OutDataTypeStr=single  SampleTime=1e-08
  Product142_pd1 : Delay  DelayLength=6
  Out1 : Outport
  wires:
  In1/1 -> Product142/1
  In2/1 -> Product142/2
  Product142/1 -> Product142_pd1/1
  Product142_pd1/1 -> Out1/1

== system gm_uz_pmsm_model/uz_pmsm_model/Product15 ==
  In1 : Inport
  In2 : Inport  Port=2
  Product15 : Product  Inputs=**  OutDataTypeStr=single  SampleTime=1e-08
  Product15_pd1 : Delay  DelayLength=6
  Out1 : Outport
  wires:
  In1/1 -> Product15/1
  In2/1 -> Product15/2
  Product15/1 -> Product15_pd1/1
  Product15_pd1/1 -> Out1/1

== system gm_uz_pmsm_model/uz_pmsm_model/Product151 ==
  In1 : Inport
  In2 : Inport  Port=2
  Product151 : Product  Inputs=**  OutDataTypeStr=single  SampleTime=1e-08
  Product151_pd1 : Delay  DelayLength=6
  Out1 : Outport
  wires:
  In1/1 -> Product151/1
  In2/1 -> Product151/2
  Product151/1 -> Product151_pd1/1
  Product151_pd1/1 -> Out1/1

== system gm_uz_pmsm_model/uz_pmsm_model/Product16 ==
  In1 : Inport
  In2 : Inport  Port=2
  Product16 : Product  Inputs=**  OutDataTypeStr=single  SampleTime=1e-08
  Product16_pd1 : Delay  DelayLength=6
  Out1 : Outport
  wires:
  In1/1 -> Product16/1
  In2/1 -> Product16/2
  Product16/1 -> Product16_pd1/1
  Product16_pd1/1 -> Out1/1

== system gm_uz_pmsm_model/uz_pmsm_model/Product17 ==
  In1 : Inport
  In2 : Inport  Port=2
  Product17 : Product  Inputs=**  OutDataTypeStr=single  SampleTime=1e-08
  Product17_pd1 : Delay  DelayLength=6
  Out1 : Outport
  wires:
  In1/1 -> Product17/1
  In2/1 -> Product17/2
  Product17/1 -> Product17_pd1/1
  Product17_pd1/1 -> Out1/1

== system gm_uz_pmsm_model/uz_pmsm_model/Product18 ==
  In1 : Inport
  In2 : Inport  Port=2
  Product18 : Product  Inputs=**  OutDataTypeStr=single  SampleTime=1e-08
  Product18_pd1 : Delay  DelayLength=6
  Out1 : Outport
  wires:
  In1/1 -> Product18/1
  In2/1 -> Product18/2
  Product18/1 -> Product18_pd1/1
  Product18_pd1/1 -> Out1/1

== system gm_uz_pmsm_model/uz_pmsm_model/Product19 ==
  In1 : Inport
  In2 : Inport  Port=2
  Product19 : Product  Inputs=**  OutDataTypeStr=single  SampleTime=1e-08
  Product19_pd1 : Delay  DelayLength=6
  Out1 : Outport
  wires:
  In1/1 -> Product19/1
  In2/1 -> Product19/2
  Product19/1 -> Product19_pd1/1
  Product19_pd1/1 -> Out1/1

== system gm_uz_pmsm_model/uz_pmsm_model/Product2 ==
  In1 : Inport
  In2 : Inport  Port=2
  Product2 : Product  Inputs=**  OutDataTypeStr=single  SampleTime=1e-08
  Product2_pd1 : Delay  DelayLength=6
  Out1 : Outport
  wires:
  In1/1 -> Product2/1
  In2/1 -> Product2/2
  Product2/1 -> Product2_pd1/1
  Product2_pd1/1 -> Out1/1

== system gm_uz_pmsm_model/uz_pmsm_model/Product20 ==
  In1 : Inport
  In2 : Inport  Port=2
  Product20 : Product  Inputs=**  OutDataTypeStr=single  SampleTime=1e-08
  Product20_pd1 : Delay  DelayLength=6
  Out1 : Outport
  wires:
  In1/1 -> Product20/1
  In2/1 -> Product20/2
  Product20/1 -> Product20_pd1/1
  Product20_pd1/1 -> Out1/1

== system gm_uz_pmsm_model/uz_pmsm_model/Product201 ==
  In1 : Inport
  In2 : Inport  Port=2
  Product201 : Product  Inputs=**  OutDataTypeStr=single  SampleTime=1e-08
  Product201_pd1 : Delay  DelayLength=6
  Out1 : Outport
  wires:
  In1/1 -> Product201/1
  In2/1 -> Product201/2
  Product201/1 -> Product201_pd1/1
  Product201_pd1/1 -> Out1/1

== system gm_uz_pmsm_model/uz_pmsm_model/Product202 ==
  In1 : Inport
  In2 : Inport  Port=2
  Product202 : Product  Inputs=**  OutDataTypeStr=single  SampleTime=1e-08
  Product202_pd1 : Delay  DelayLength=6
  Out1 : Outport
  wires:
  In1/1 -> Product202/1
  In2/1 -> Product202/2
  Product202/1 -> Product202_pd1/1
  Product202_pd1/1 -> Out1/1

== system gm_uz_pmsm_model/uz_pmsm_model/Product203 ==
  In1 : Inport
  In2 : Inport  Port=2
  Product203 : Product  Inputs=**  OutDataTypeStr=single  SampleTime=1e-08
  Product203_pd1 : Delay  DelayLength=6
  Out1 : Outport
  wires:
  In1/1 -> Product203/1
  In2/1 -> Product203/2
  Product203/1 -> Product203_pd1/1
  Product203_pd1/1 -> Out1/1

== system gm_uz_pmsm_model/uz_pmsm_model/Product204 ==
  In1 : Inport
  In2 : Inport  Port=2
  Product204 : Product  Inputs=**  OutDataTypeStr=single  SampleTime=1e-08
  Product204_pd1 : Delay  DelayLength=6
  Out1 : Outport
  wires:
  In1/1 -> Product204/1
  In2/1 -> Product204/2
  Product204/1 -> Product204_pd1/1
  Product204_pd1/1 -> Out1/1

== system gm_uz_pmsm_model/uz_pmsm_model/Product205 ==
  In1 : Inport
  In2 : Inport  Port=2
  Product205 : Product  Inputs=**  OutDataTypeStr=single  SampleTime=1e-08
  Product205_pd1 : Delay  DelayLength=6
  Out1 : Outport
  wires:
  In1/1 -> Product205/1
  In2/1 -> Product205/2
  Product205/1 -> Product205_pd1/1
  Product205_pd1/1 -> Out1/1

== system gm_uz_pmsm_model/uz_pmsm_model/Product206 ==
  In1 : Inport
  In2 : Inport  Port=2
  Product206 : Product  Inputs=**  OutDataTypeStr=single  SampleTime=1e-08
  Product206_pd1 : Delay  DelayLength=6
  Out1 : Outport
  wires:
  In1/1 -> Product206/1
  In2/1 -> Product206/2
  Product206/1 -> Product206_pd1/1
  Product206_pd1/1 -> Out1/1

== system gm_uz_pmsm_model/uz_pmsm_model/Product207 ==
  In1 : Inport
  In2 : Inport  Port=2
  Product207 : Product  Inputs=**  OutDataTypeStr=single  SampleTime=1e-08
  Product207_pd1 : Delay  DelayLength=6
  Out1 : Outport
  wires:
  In1/1 -> Product207/1
  In2/1 -> Product207/2
  Product207/1 -> Product207_pd1/1
  Product207_pd1/1 -> Out1/1

== system gm_uz_pmsm_model/uz_pmsm_model/Product21 ==
  In1 : Inport
  In2 : Inport  Port=2
  Product21 : Product  Inputs=**  OutDataTypeStr=single  SampleTime=1e-08
  Product21_pd1 : Delay  DelayLength=6
  Out1 : Outport
  wires:
  In1/1 -> Product21/1
  In2/1 -> Product21/2
  Product21/1 -> Product21_pd1/1
  Product21_pd1/1 -> Out1/1

== system gm_uz_pmsm_model/uz_pmsm_model/Product22 ==
  In1 : Inport
  In2 : Inport  Port=2
  Product22 : Product  Inputs=**  OutDataTypeStr=single  SampleTime=1e-08
  Product22_pd1 : Delay  DelayLength=6
  Out1 : Outport
  wires:
  In1/1 -> Product22/1
  In2/1 -> Product22/2
  Product22/1 -> Product22_pd1/1
  Product22_pd1/1 -> Out1/1

== system gm_uz_pmsm_model/uz_pmsm_model/Product23 ==
  In1 : Inport
  In2 : Inport  Port=2
  Product23 : Product  Inputs=**  OutDataTypeStr=single  SampleTime=1e-08
  Product23_pd1 : Delay  DelayLength=6
  Out1 : Outport
  wires:
  In1/1 -> Product23/1
  In2/1 -> Product23/2
  Product23/1 -> Product23_pd1/1
  Product23_pd1/1 -> Out1/1

== system gm_uz_pmsm_model/uz_pmsm_model/Product24 ==
  In1 : Inport
  In2 : Inport  Port=2
  Product24 : Product  Inputs=**  OutDataTypeStr=single  SampleTime=1e-08
  Product24_pd1 : Delay  DelayLength=6
  Out1 : Outport
  wires:
  In1/1 -> Product24/1
  In2/1 -> Product24/2
  Product24/1 -> Product24_pd1/1
  Product24_pd1/1 -> Out1/1

== system gm_uz_pmsm_model/uz_pmsm_model/Product25 ==
  In1 : Inport
  In2 : Inport  Port=2
  Product25 : Product  Inputs=**  OutDataTypeStr=single  SampleTime=1e-08
  Product25_pd1 : Delay  DelayLength=6
  Out1 : Outport
  wires:
  In1/1 -> Product25/1
  In2/1 -> Product25/2
  Product25/1 -> Product25_pd1/1
  Product25_pd1/1 -> Out1/1

== system gm_uz_pmsm_model/uz_pmsm_model/Product3 ==
  In1 : Inport
  In2 : Inport  Port=2
  Product3 : Product  Inputs=**  OutDataTypeStr=single  SampleTime=1e-08
  Product3_pd1 : Delay  DelayLength=6
  Out1 : Outport
  wires:
  In1/1 -> Product3/1
  In2/1 -> Product3/2
  Product3/1 -> Product3_pd1/1
  Product3_pd1/1 -> Out1/1

== system gm_uz_pmsm_model/uz_pmsm_model/Product31 ==
  In1 : Inport
  In2 : Inport  Port=2
  Product31 : Product  Inputs=**  OutDataTypeStr=single  SampleTime=1e-08
  Product31_pd1 : Delay  DelayLength=6
  Out1 : Outport
  wires:
  In1/1 -> Product31/1
  In2/1 -> Product31/2
  Product31/1 -> Product31_pd1/1
  Product31_pd1/1 -> Out1/1

== system gm_uz_pmsm_model/uz_pmsm_model/Product32 ==
  In1 : Inport
  In2 : Inport  Port=2
  Product32 : Product  Inputs=**  OutDataTypeStr=single  SampleTime=1e-08
  Product32_pd1 : Delay  DelayLength=6
  Out1 : Outport
  wires:
  In1/1 -> Product32/1
  In2/1 -> Product32/2
  Product32/1 -> Product32_pd1/1
  Product32_pd1/1 -> Out1/1

== system gm_uz_pmsm_model/uz_pmsm_model/Product33 ==
  In1 : Inport
  In2 : Inport  Port=2
  Product33 : Product  Inputs=**  OutDataTypeStr=single  SampleTime=1e-08
  Product33_pd1 : Delay  DelayLength=6
  Out1 : Outport
  wires:
  In1/1 -> Product33/1
  In2/1 -> Product33/2
  Product33/1 -> Product33_pd1/1
  Product33_pd1/1 -> Out1/1

== system gm_uz_pmsm_model/uz_pmsm_model/Product34 ==
  In1 : Inport
  In2 : Inport  Port=2
  Product34 : Product  Inputs=**  OutDataTypeStr=single  SampleTime=1e-08
  Product34_pd1 : Delay  DelayLength=6
  Out1 : Outport
  wires:
  In1/1 -> Product34/1
  In2/1 -> Product34/2
  Product34/1 -> Product34_pd1/1
  Product34_pd1/1 -> Out1/1

== system gm_uz_pmsm_model/uz_pmsm_model/Product35 ==
  In1 : Inport
  In2 : Inport  Port=2
  Product35 : Product  Inputs=**  OutDataTypeStr=single  SampleTime=1e-08
  Product35_pd1 : Delay  DelayLength=6
  Out1 : Outport
  wires:
  In1/1 -> Product35/1
  In2/1 -> Product35/2
  Product35/1 -> Product35_pd1/1
  Product35_pd1/1 -> Out1/1

== system gm_uz_pmsm_model/uz_pmsm_model/Product4 ==
  In1 : Inport
  In2 : Inport  Port=2
  Product4 : Product  Inputs=**  OutDataTypeStr=single  SampleTime=1e-08
  Product4_pd1 : Delay  DelayLength=6
  Out1 : Outport
  wires:
  In1/1 -> Product4/1
  In2/1 -> Product4/2
  Product4/1 -> Product4_pd1/1
  Product4_pd1/1 -> Out1/1

== system gm_uz_pmsm_model/uz_pmsm_model/Product41 ==
  In1 : Inport
  In2 : Inport  Port=2
  Product41 : Product  Inputs=**  OutDataTypeStr=single  SampleTime=1e-08
  Product41_pd1 : Delay  DelayLength=6
  Out1 : Outport
  wires:
  In1/1 -> Product41/1
  In2/1 -> Product41/2
  Product41/1 -> Product41_pd1/1
  Product41_pd1/1 -> Out1/1

== system gm_uz_pmsm_model/uz_pmsm_model/Product42 ==
  In1 : Inport
  In2 : Inport  Port=2
  Product42 : Product  Inputs=**  OutDataTypeStr=single  SampleTime=1e-08
  Product42_pd1 : Delay  DelayLength=6
  Out1 : Outport
  wires:
  In1/1 -> Product42/1
  In2/1 -> Product42/2
  Product42/1 -> Product42_pd1/1
  Product42_pd1/1 -> Out1/1

== system gm_uz_pmsm_model/uz_pmsm_model/Product43 ==
  In1 : Inport
  In2 : Inport  Port=2
  Product43 : Product  Inputs=**  OutDataTypeStr=single  SampleTime=1e-08
  Product43_pd1 : Delay  DelayLength=6
  Out1 : Outport
  wires:
  In1/1 -> Product43/1
  In2/1 -> Product43/2
  Product43/1 -> Product43_pd1/1
  Product43_pd1/1 -> Out1/1

== system gm_uz_pmsm_model/uz_pmsm_model/Product5 ==
  In1 : Inport
  In2 : Inport  Port=2
  Product5 : Product  Inputs=**  OutDataTypeStr=single  SampleTime=1e-08
  Product5_pd1 : Delay  DelayLength=6
  Out1 : Outport
  wires:
  In1/1 -> Product5/1
  In2/1 -> Product5/2
  Product5/1 -> Product5_pd1/1
  Product5_pd1/1 -> Out1/1

== system gm_uz_pmsm_model/uz_pmsm_model/Product51 ==
  In1 : Inport
  In2 : Inport  Port=2
  Product51 : Product  Inputs=**  OutDataTypeStr=single  SampleTime=1e-08
  Product51_pd1 : Delay  DelayLength=6
  Out1 : Outport
  wires:
  In1/1 -> Product51/1
  In2/1 -> Product51/2
  Product51/1 -> Product51_pd1/1
  Product51_pd1/1 -> Out1/1

== system gm_uz_pmsm_model/uz_pmsm_model/Product52 ==
  In1 : Inport
  In2 : Inport  Port=2
  Product52 : Product  Inputs=**  OutDataTypeStr=single  SampleTime=1e-08
  Product52_pd1 : Delay  DelayLength=6
  Out1 : Outport
  wires:
  In1/1 -> Product52/1
  In2/1 -> Product52/2
  Product52/1 -> Product52_pd1/1
  Product52_pd1/1 -> Out1/1

== system gm_uz_pmsm_model/uz_pmsm_model/Product6 ==
  In1 : Inport
  In2 : Inport  Port=2
  Product6 : Product  Inputs=**  OutDataTypeStr=single  SampleTime=1e-08
  Product6_pd1 : Delay  DelayLength=6
  Out1 : Outport
  wires:
  In1/1 -> Product6/1
  In2/1 -> Product6/2
  Product6/1 -> Product6_pd1/1
  Product6_pd1/1 -> Out1/1

== system gm_uz_pmsm_model/uz_pmsm_model/Product61 ==
  In1 : Inport
  In2 : Inport  Port=2
  Product61 : Product  Inputs=**  OutDataTypeStr=single  SampleTime=1e-08
  Product61_pd1 : Delay  DelayLength=6
  Out1 : Outport
  wires:
  In1/1 -> Product61/1
  In2/1 -> Product61/2
  Product61/1 -> Product61_pd1/1
  Product61_pd1/1 -> Out1/1

== system gm_uz_pmsm_model/uz_pmsm_model/Product7 ==
  In1 : Inport
  In2 : Inport  Port=2
  Product7 : Product  Inputs=**  OutDataTypeStr=single  SampleTime=1e-08
  Product7_pd1 : Delay  DelayLength=6
  Out1 : Outport
  wires:
  In1/1 -> Product7/1
  In2/1 -> Product7/2
  Product7/1 -> Product7_pd1/1
  Product7_pd1/1 -> Out1/1

== system gm_uz_pmsm_model/uz_pmsm_model/Product71 ==
  In1 : Inport
  In2 : Inport  Port=2
  Product71 : Product  Inputs=**  OutDataTypeStr=single  SampleTime=1e-08
  Product71_pd1 : Delay  DelayLength=6
  Out1 : Outport
  wires:
  In1/1 -> Product71/1
  In2/1 -> Product71/2
  Product71/1 -> Product71_pd1/1
  Product71_pd1/1 -> Out1/1

== system gm_uz_pmsm_model/uz_pmsm_model/Product8 ==
  In1 : Inport
  In2 : Inport  Port=2
  Product8 : Product  Inputs=**  OutDataTypeStr=single  SampleTime=1e-08
  Product8_pd1 : Delay  DelayLength=6
  Out1 : Outport
  wires:
  In1/1 -> Product8/1
  In2/1 -> Product8/2
  Product8/1 -> Product8_pd1/1
  Product8_pd1/1 -> Out1/1

== system gm_uz_pmsm_model/uz_pmsm_model/Product9 ==
  In1 : Inport
  In2 : Inport  Port=2
  Product9 : Product  Inputs=**  OutDataTypeStr=single  SampleTime=1e-08
  Product9_pd1 : Delay  DelayLength=6
  Out1 : Outport
  wires:
  In1/1 -> Product9/1
  In2/1 -> Product9/2
  Product9/1 -> Product9_pd1/1
  Product9_pd1/1 -> Out1/1

== system gm_uz_pmsm_model/uz_pmsm_model/Product91 ==
  In1 : Inport
  In2 : Inport  Port=2
  Product91 : Product  Inputs=**  OutDataTypeStr=single  SampleTime=1e-08
  Product91_pd1 : Delay  DelayLength=6
  Out1 : Outport
  wires:
  In1/1 -> Product91/1
  In2/1 -> Product91/2
  Product91/1 -> Product91_pd1/1
  Product91_pd1/1 -> Out1/1

== system gm_uz_pmsm_model/uz_pmsm_model/Product92 ==
  In1 : Inport
  In2 : Inport  Port=2
  Product92 : Product  Inputs=**  OutDataTypeStr=single  SampleTime=1e-08
  Product92_pd1 : Delay  DelayLength=6
  Out1 : Outport
  wires:
  In1/1 -> Product92/1
  In2/1 -> Product92/2
  Product92/1 -> Product92_pd1/1
  Product92_pd1/1 -> Out1/1

== system gm_uz_pmsm_model/uz_pmsm_model/Reciprocal1_recip ==
  In1 : Inport
  Reciprocal1_recip : Math  Operator=reciprocal  SampleTime=1e-08
  Reciprocal1_recip_pd1 : Delay  DelayLength=16
  Out1 : Outport
  wires:
  In1/1 -> Reciprocal1_recip/1
  Reciprocal1_recip/1 -> Reciprocal1_recip_pd1/1
  Reciprocal1_recip_pd1/1 -> Out1/1

== system gm_uz_pmsm_model/uz_pmsm_model/Reciprocal1_recip1 ==
  In1 : Inport
  Reciprocal1_recip1 : Math  Operator=reciprocal  SampleTime=1e-08
  Reciprocal1_recip1_pd1 : Delay  DelayLength=16
  Out1 : Outport
  wires:
  In1/1 -> Reciprocal1_recip1/1
  Reciprocal1_recip1/1 -> Reciprocal1_recip1_pd1/1
  Reciprocal1_recip1_pd1/1 -> Out1/1

== system gm_uz_pmsm_model/uz_pmsm_model/Reciprocal_recip ==
  In1 : Inport
  Reciprocal_recip : Math  Operator=reciprocal  SampleTime=1e-08
  Reciprocal_recip_pd1 : Delay  DelayLength=16
  Out1 : Outport
  wires:
  In1/1 -> Reciprocal_recip/1
  Reciprocal_recip/1 -> Reciprocal_recip_pd1/1
  Reciprocal_recip_pd1/1 -> Out1/1

== system gm_uz_pmsm_model/uz_pmsm_model/Reciprocal_recip1 ==
  In1 : Inport
  Reciprocal_recip1 : Math  Operator=reciprocal  SampleTime=1e-08
  Reciprocal_recip1_pd1 : Delay  DelayLength=16
  Out1 : Outport
  wires:
  In1/1 -> Reciprocal_recip1/1
  Reciprocal_recip1/1 -> Reciprocal_recip1_pd1/1
  Reciprocal_recip1_pd1/1 -> Out1/1

== system gm_uz_pmsm_model/uz_pmsm_model/Sign1 ==
  In1 : Inport
  Sign1 : Signum  SampleTime=1e-08
  Out1 : Outport
  wires:
  In1/1 -> Sign1/1
  Sign1/1 -> Out1/1

== system gm_uz_pmsm_model/uz_pmsm_model/Sum ==
  In1 : Inport
  In2 : Inport  Port=2
  Sum : Sum  OutDataTypeStr=single  SampleTime=1e-08
  Sum_pd1 : Delay  DelayLength=6
  Out1 : Outport
  wires:
  In1/1 -> Sum/1
  In2/1 -> Sum/2
  Sum/1 -> Sum_pd1/1
  Sum_pd1/1 -> Out1/1

== system gm_uz_pmsm_model/uz_pmsm_model/Sum1 ==
  In1 : Inport
  In2 : Inport  Port=2
  Sum1 : Sum  Inputs=+-  OutDataTypeStr=single  SampleTime=1e-08
  Sum1_pd1 : Delay  DelayLength=6
  Out1 : Outport
  wires:
  In1/1 -> Sum1/1
  In2/1 -> Sum1/2
  Sum1/1 -> Sum1_pd1/1
  Sum1_pd1/1 -> Out1/1

== system gm_uz_pmsm_model/uz_pmsm_model/Sum10 ==
  In1 : Inport
  In2 : Inport  Port=2
  Sum10 : Sum  Inputs=+-  OutDataTypeStr=single  SampleTime=1e-08
  Sum10_pd1 : Delay  DelayLength=6
  Out1 : Outport
  wires:
  In1/1 -> Sum10/1
  In2/1 -> Sum10/2
  Sum10/1 -> Sum10_pd1/1
  Sum10_pd1/1 -> Out1/1

== system gm_uz_pmsm_model/uz_pmsm_model/Sum101 ==
  In1 : Inport
  In2 : Inport  Port=2
  Sum101 : Sum  Inputs=+-  OutDataTypeStr=single  SampleTime=1e-08
  Sum101_pd1 : Delay  DelayLength=6
  Out1 : Outport
  wires:
  In1/1 -> Sum101/1
  In2/1 -> Sum101/2
  Sum101/1 -> Sum101_pd1/1
  Sum101_pd1/1 -> Out1/1

== system gm_uz_pmsm_model/uz_pmsm_model/Sum11 ==
  In1 : Inport
  In2 : Inport  Port=2
  Sum11 : Sum  Inputs=+-  OutDataTypeStr=single  SampleTime=1e-08
  Sum11_pd1 : Delay  DelayLength=6
  Out1 : Outport
  wires:
  In1/1 -> Sum11/1
  In2/1 -> Sum11/2
  Sum11/1 -> Sum11_pd1/1
  Sum11_pd1/1 -> Out1/1

== system gm_uz_pmsm_model/uz_pmsm_model/Sum12 ==
  In1 : Inport
  In2 : Inport  Port=2
  Sum12 : Sum  OutDataTypeStr=single  SampleTime=1e-08
  Sum12_pd1 : Delay  DelayLength=6
  Out1 : Outport
  wires:
  In1/1 -> Sum12/1
  In2/1 -> Sum12/2
  Sum12/1 -> Sum12_pd1/1
  Sum12_pd1/1 -> Out1/1

== system gm_uz_pmsm_model/uz_pmsm_model/Sum13 ==
  In1 : Inport
  In2 : Inport  Port=2
  Sum13 : Sum  OutDataTypeStr=single  SampleTime=1e-08
  Sum13_pd1 : Delay  DelayLength=6
  Out1 : Outport
  wires:
  In1/1 -> Sum13/1
  In2/1 -> Sum13/2
  Sum13/1 -> Sum13_pd1/1
  Sum13_pd1/1 -> Out1/1

== system gm_uz_pmsm_model/uz_pmsm_model/Sum14 ==
  In1 : Inport
  In2 : Inport  Port=2
  Sum14 : Sum  Inputs=+-  OutDataTypeStr=single  SampleTime=1e-08
  Sum14_pd1 : Delay  DelayLength=6
  Out1 : Outport
  wires:
  In1/1 -> Sum14/1
  In2/1 -> Sum14/2
  Sum14/1 -> Sum14_pd1/1
  Sum14_pd1/1 -> Out1/1

== system gm_uz_pmsm_model/uz_pmsm_model/Sum2 ==
  In1 : Inport
  In2 : Inport  Port=2
  Sum2 : Sum  Inputs=+-  OutDataTypeStr=single  SampleTime=1e-08
  Sum2_pd1 : Delay  DelayLength=6
  Out1 : Outport
  wires:
  In1/1 -> Sum2/1
  In2/1 -> Sum2/2
  Sum2/1 -> Sum2_pd1/1
  Sum2_pd1/1 -> Out1/1

== system gm_uz_pmsm_model/uz_pmsm_model/Sum21 ==
  In1 : Inport
  In2 : Inport  Port=2
  Sum21 : Sum  Inputs=+-  OutDataTypeStr=single  SampleTime=1e-08
  Sum21_pd1 : Delay  DelayLength=6
  Out1 : Outport
  wires:
  In1/1 -> Sum21/1
  In2/1 -> Sum21/2
  Sum21/1 -> Sum21_pd1/1
  Sum21_pd1/1 -> Out1/1

== system gm_uz_pmsm_model/uz_pmsm_model/Sum22 ==
  In1 : Inport
  In2 : Inport  Port=2
  Sum22 : Sum  Inputs=+-  OutDataTypeStr=single  SampleTime=1e-08
  Sum22_pd1 : Delay  DelayLength=6
  Out1 : Outport
  wires:
  In1/1 -> Sum22/1
  In2/1 -> Sum22/2
  Sum22/1 -> Sum22_pd1/1
  Sum22_pd1/1 -> Out1/1
